simulink model "Statechart_Destructeur_Aiguille"  (R2023a)
settings: Solver=FixedStepAuto  StartTime=0.0  StopTime=inf  FixedStep=0.0005  RelTol=1e-3  EnableMultiTasking=on
libraries: arduinolib x10
settings Model: ExtModeTrigDuration=2  Creator=Renaud  LastModifiedBy=renaud.costadoat
settings SolverCC: AlgebraicLoopSolver=TrustRegion
settings OptimizationCC: EnhancedBackFolding=on  PassReuseOutputArgsAs=Individual arguments  ZeroExternalMemoryAtStartup=off  ZeroInternalMemoryAtStartup=off  MaxStackSize=64  OptimizeBlockOrder=speed  DifferentSizesBufferReuse=on  OptimizationCustomize=off  EfficientTunableParamExpr=on
settings DebuggingCC: ParameterTunabilityLossMsg=error  UnconnectedInputMsg=warning  UnconnectedOutputMsg=warning  UnconnectedLineMsg=warning
settings HardwareCC: ProdBitPerInt=16  ProdBitPerPointer=16  ProdBitPerSizeT=16  ProdBitPerPtrDiffT=16  ProdLargestAtomicFloat=None  ProdWordSize=8  ProdHWDeviceType=Atmel->AVR
settings ModelReferenceCC: EnableRefExpFcnMdlSchedulingChecks=on
settings SFSimCC: MATLABDynamicMemAlloc=off
settings RTWCC: Description=Embedded Coder  SystemTargetFile=ert.tlc  HardwareBoard=Arduino Uno  TemplateMakefile=ert_default_tmf  Toolchain=Arduino AVR  BuildConfiguration=Faster Runs
settings CodeAppCC: ForceParamTrailComments=on  IgnoreCustomStorageClasses=off  OperatorAnnotations=on  SimulinkDataObjDesc=on  SFDataObjDesc=on  InsertBlockDesc=on
settings ERTTargetCC: SupportContinuousTime=on  SupportVariableSizeSignals=on  ExtModeTransport=3  ExtModeStaticAlloc=on  ExtModeAutomaticAllocSize=off  ExtModeStaticAllocSize=250  ExtModeMexFile=ext_xcp  ExtModeIntrfLevel=Level2 - Open

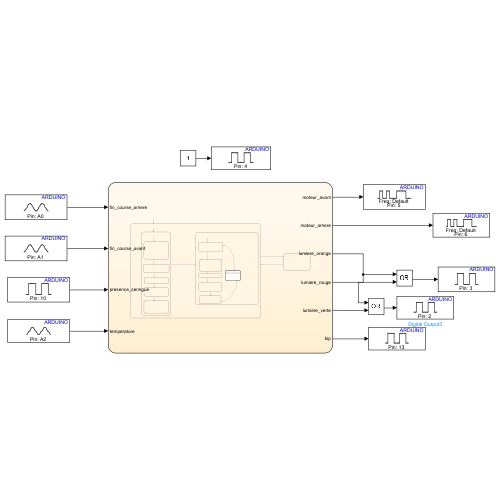
[thumbnail: Simulink's stored preview of the top-level diagram]
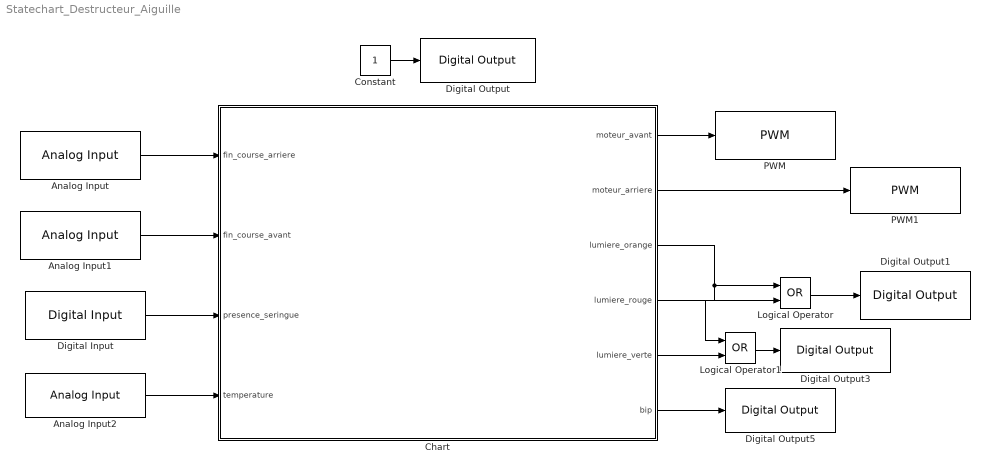
== system Statechart_Destructeur_Aiguille ==
  Analog Input : arduinolib/Analog Input  pinNumber=0  ReadResultsOnly=off  ConversionTriggerSource=Software  ExternalTriggerType=uint32( 0 )  OutputDataType=uint16  EnableConversionCompleteNotify=off  EnableOuputStatus=off  SampleTime=-1  blockPlatform=arduino
  Analog Input1 : arduinolib/Analog Input  pinNumber=1  ReadResultsOnly=off  ConversionTriggerSource=Software  ExternalTriggerType=uint32( 0 )  OutputDataType=uint16  EnableConversionCompleteNotify=off  EnableOuputStatus=off  SampleTime=-1  blockPlatform=arduino
  Analog Input2 : arduinolib/Analog Input  pinNumber=2  ReadResultsOnly=off  ConversionTriggerSource=Software  ExternalTriggerType=uint32( 0 )  OutputDataType=uint16  EnableConversionCompleteNotify=off  EnableOuputStatus=off  SampleTime=-1  blockPlatform=arduino
  Chart : Stateflow chart  TreatAsAtomicUnit=on
  Constant : Constant
  Digital Input : arduinolib/Digital Input  pinNumber=10  mode=Default  Direction=input  SampleTime=-1  blockPlatform=arduino
  Digital Output : arduinolib/Digital Output  pinNumber=4  Direction=output  blockPlatform=arduino
  Digital Output1 : arduinolib/Digital Output  pinNumber=3  Direction=output  blockPlatform=arduino
  Digital Output3 : arduinolib/Digital Output  pinNumber=2  Direction=output  blockPlatform=arduino
  Digital Output5 : arduinolib/Digital Output  pinNumber=13  Direction=output  blockPlatform=arduino
  Logical Operator : Logic  Operator=OR  AllPortsSameDT=off  OutDataTypeStr=boolean
  Logical Operator1 : Logic  Operator=OR  AllPortsSameDT=off  OutDataTypeStr=boolean
  PWM : arduinolib/PWM  pinNumber=5  frequencyType=Default  desiredFrequency=490.2  achievableFrequency=490.2
  PWM1 : arduinolib/PWM  pinNumber=6  frequencyType=Default  desiredFrequency=490.2  achievableFrequency=490.2
  wires:
  Chart/1(moteur_avant) -> PWM/1
  Analog Input1/1 -> Chart/2(fin_course_avant)
  Analog Input2/1 -> Chart/4(temperature)
  Digital Input/1 -> Chart/3(presence_seringue)
  Chart/2(moteur_arriere) -> PWM1/1
  Logical Operator/1 -> Digital Output1/1
  Chart/3(lumiere_orange) -> Logical Operator1/1, Logical Operator/1
  Chart/4(lumiere_rouge) -> Logical Operator/2
  Logical Operator1/1 -> Digital Output3/1
  Chart/5(lumiere_verte) -> Logical Operator1/2
  Chart/6(bip) -> Digital Output5/1
  Constant/1 -> Digital Output/1
  Analog Input/1 -> Chart/1(fin_course_arriere)

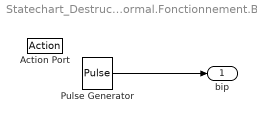
== system Statechart_Destructeur_Aiguille/Chart/Fonctionnement_normal.Fonctionnement.Beep ==
  Action Port : ActionPort
      settings: CopyFcn=Stateflow.SLINSF.SimulinkMan.removeBlockPreDeleteFcn  PreDeleteFcn=Stateflow.SLINSF.SimulinkMan.unsafePredeleteFcn
  Pulse Generator : DiscretePulseGenerator  PulseType=Time based  Amplitude=1024  Period=0.002  PulseWidth=50
  bip : Outport
  wires:
  Pulse Generator/1 -> bip/1

== stateflow chart Statechart_Destructeur_Aiguille/Chart ==
  state Fonctionnement_normal
    state Initialisation
      state Attente_initialisation
        entry:machine_prete=0
        entry:moteur_avant=0
        entry:moteur_arriere=0
        entry:lumiere_verte=0
        entry:lumiere_rouge=0
        entry:lumiere_orange=1
      state Avancer_lame
        entry:moteur_avant=200
        exit:moteur_avant=0
      state Attente
      state Reculer_lame
        entry:moteur_arriere=200
        exit:moteur_arriere=0
      state Attente1
        entry:bip=1
        entry:machine_prete=1
        entry:lumiere_orange=0
        exit:bip=0
      (default) -> Attente_initialisation
      Attente_initialisation -> Avancer_lame : after(0.5,sec)
      Avancer_lame -> Fonctionnement_normal.Initialisation.Attente : after(0.5,sec)
      Fonctionnement_normal.Initialisation.Attente -> Reculer_lame : after(1,sec)
      Reculer_lame -> Fonctionnement_normal.Initialisation.Attente1 : after(0.5,sec)
    state Fonctionnement
      state Attente_serringue
        entry:lumiere_verte=1
        exit:lumiere_verte=0
      state Avance_lame
        entry:moteur_avant=200
        entry:moteur_arriere=0
        entry:lumiere_orange=1
        exit:moteur_avant=0
      state Beep
      state Attente
      state Recul_lame
        entry:moteur_avant=0
        entry:moteur_arriere=200
        exit:moteur_arriere=0
      state Attente1
        entry:lumiere_orange=0
        entry:lumiere_verte=1
      (default) -> Attente_serringue
      Beep -> Attente_serringue : after(1,sec)
      Attente_serringue -> Avance_lame : [presence_seringue==1]
      Avance_lame -> Fonctionnement_normal.Fonctionnement.Attente : after(0.4,sec)
      Fonctionnement_normal.Fonctionnement.Attente -> Recul_lame : after(0.1,sec)
      Fonctionnement_normal.Fonctionnement.Attente1 -> Beep : [presence_seringue==0]
      Recul_lame -> Fonctionnement_normal.Fonctionnement.Attente1 : after(0.4,sec)
    (default) -> Initialisation
    Initialisation -> Fonctionnement : [machine_prete==1]
  state Erreur
    entry: lumiere_verte=0
    entry: lumiere_orange=0
    entry: lumiere_rouge=1
    entry: machine_prete=0
    exit: lumiere_rouge=0
  (default) -> Fonctionnement_normal
  Fonctionnement_normal -> Erreur : [temperature>1000]
  Erreur -> Fonctionnement_normal : [temperature<800]
  data: sf_internal_action_state_placeholder_data local double size=1 =0; moteur_avant output; moteur_arriere output; fin_course_arriere input; fin_course_avant input; presence_seringue input; lumiere_orange output; lumiere_rouge output; lumiere_verte output; bip output; machine_prete local =0; temperature input
